simulink model "testXY"  (Simulink 7.9)
settings: Solver=ode3  StartTime=0.0  StopTime=10.0  FixedStep=sampleTs/100  RelTol=1e-3
values from neighbouring files (symbols this model uses):
  Bd1 = Adtemp*(Bdt)    [tuneXYControl.m]    (also in tuneZControl.m)
  Bd2 = Bdt    [tuneXYControl.m]    (also in tuneZControl.m)
  delay = delay + 0.14    (= 0.14)    [tuneXYControl.m]    (also in tuneZControl.m = 0.18)
  Kc = dlqr(SSD.a,SSD.b,QR,RR)    [tuneXYControl.m]    (also in tuneZControl.m)
  Lc2 = dlqe(Ad,Bd,Cd,inputNoise*inputNoise,RE)    [tuneXYControl.m]    (also in tuneZControl.m)
  matErrA = 1.0    (= 1)    [tuneXYControl.m]    (also in tuneZControl.m)
  matErrB = 1.0    (= 1)    [tuneXYControl.m]    (also in tuneZControl.m)
  matErrC = 1.0    (= 1)    [tuneXYControl.m]    (also in tuneZControl.m)
  n = n+1    (= 1)    [tuneXYControl.m]    (also in tuneZControl.m)
  ssc = ss(Ac,Bc,Cc,Dc)    [tuneXYControl.m]    (also in tuneZControl.m)
  stepDist = 0.2    [tuneXYControl.m]    (also in tuneZControl.m = 0.1)
undefined symbols (not defined in the file or in its folder): Ad, Cd
libraries: simulink x1
settings Model: Creator=user  LastModifiedBy=user
settings GRTTargetCC: CombineOutputUpdateFcns=off  GRTInterface=on

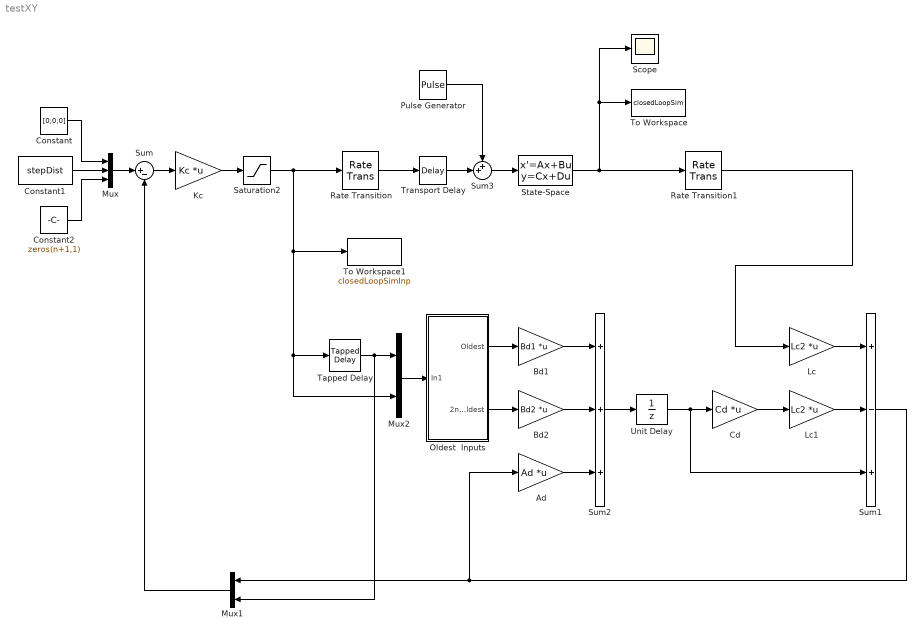
== system testXY ==
  Ad : Gain  Gain=Ad  Multiplication=Matrix(K*u)
  Bd1 : Gain  Gain=Bd1  Multiplication=Matrix(K*u)
  Bd2 : Gain  Gain=Bd2  Multiplication=Matrix(K*u)
  Cd : Gain  Gain=Cd  Multiplication=Matrix(K*u)
  Constant : Constant  Value=[0;0;0]
  Constant1 : Constant  Value=stepDist
  Constant2 : Constant  Value=zeros(n+1,1)
  Kc : Gain  Gain=Kc  Multiplication=Matrix(K*u)
  Lc : Gain  Gain=Lc2  Multiplication=Matrix(K*u)
  Lc1 : Gain  Gain=Lc2  Multiplication=Matrix(K*u)
  Mux : Mux  Inputs=3
  Mux1 : Mux  Inputs=2
  Mux2 : Mux  Inputs=2
  Oldest  Inputs : Subsystem
  Pulse Generator : DiscretePulseGenerator  PulseType=Time based  Amplitude=-stepDist*3.0  Period=100  PulseWidth=0.1  PhaseDelay=5.0
  Rate Transition : RateTransition  Deterministic=off
  Rate Transition1 : RateTransition  Deterministic=off  OutPortSampleTime=sampleTs
  Saturation2 : Saturate  UpperLimit=0.37  LowerLimit=-0.37
  Scope : Scope
  State-Space : StateSpace  A=matErrA*ssc.a  B=matErrB*ssc.b  C=matErrC*ssc.c  D=ssc.d
  Sum : Sum  Inputs=|+-
  Sum1 : Sum  Inputs=+-+
  Sum2 : Sum  Inputs=+++
  Sum3 : Sum  Inputs=++|
  Tapped Delay : simulink/Discrete/Tapped Delay  vinit=0  samptime=sampleTs  NumDelays=n+1  DelayOrder=Oldest  includeCurrent=off
  To Workspace : ToWorkspace  VariableName=closedLoopSim  SampleTime=-1  SaveFormat=Structure With Time
  To Workspace1 : ToWorkspace  VariableName=closedLoopSimInp  SampleTime=-1  SaveFormat=Structure With Time
  Transport Delay : TransportDelay  DelayTime=delay  BufferSize=4096
  Unit Delay : UnitDelay  SampleTime=-1
  wires:
  Constant/1 -> Mux/1
  Constant1/1 -> Mux/2
  Constant2/1 -> Mux/3
  Mux/1 -> Sum/1
  Rate Transition/1 -> Transport Delay/1
  State-Space/1 -> Rate Transition1/1, Scope/1, To Workspace/1
  Rate Transition1/1 -> Lc/1
  Lc/1 -> Sum1/1
  Lc1/1 -> Sum1/2
  Cd/1 -> Lc1/1
  Unit Delay/1 -> Cd/1, Sum1/3
  Sum1/1 -> Mux1/1, Ad/1
  Sum2/1 -> Unit Delay/1
  Sum/1 -> Kc/1
  Ad/1 -> Sum2/3
  Bd2/1 -> Sum2/2
  Bd1/1 -> Sum2/1
  Mux1/1 -> Sum/2
  Oldest  Inputs/1(Oldest) -> Bd1/1
  Oldest  Inputs/2(2ndOldest) -> Bd2/1
  Mux2/1 -> Oldest  Inputs/1(In1)
  Tapped Delay/1 -> Mux2/1, Mux1/2
  Kc/1 -> Saturation2/1
  Saturation2/1 -> Rate Transition/1, Tapped Delay/1, Mux2/2, To Workspace1/1
  Sum3/1 -> State-Space/1
  Transport Delay/1 -> Sum3/2
  Pulse Generator/1 -> Sum3/1

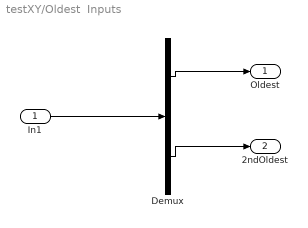
== system testXY/Oldest  Inputs ==
  In1 : Inport
  Demux : Demux  Outputs=n+2
  Oldest : Outport
  2ndOldest : Outport  Port=2
  wires:
  Demux/1 -> Oldest/1
  Demux/2 -> 2ndOldest/1
  In1/1 -> Demux/1
